simulink model "Three_Phase_SPWM_Boost_Rectifier2015b"  (Simulink 8.6)
settings: Solver=ode45  StartTime=0.0  StopTime=0.8  RelTol=1e-3
libraries: powerlib x20, simulink x4, powerlib_meascontrol x3
settings Model: Creator=sample  LastModifiedBy=A0109971
settings DebuggingCC: FcnCallInpInsideContextMsg=EnableAllAsWarning  AllowSymbolicDim=on

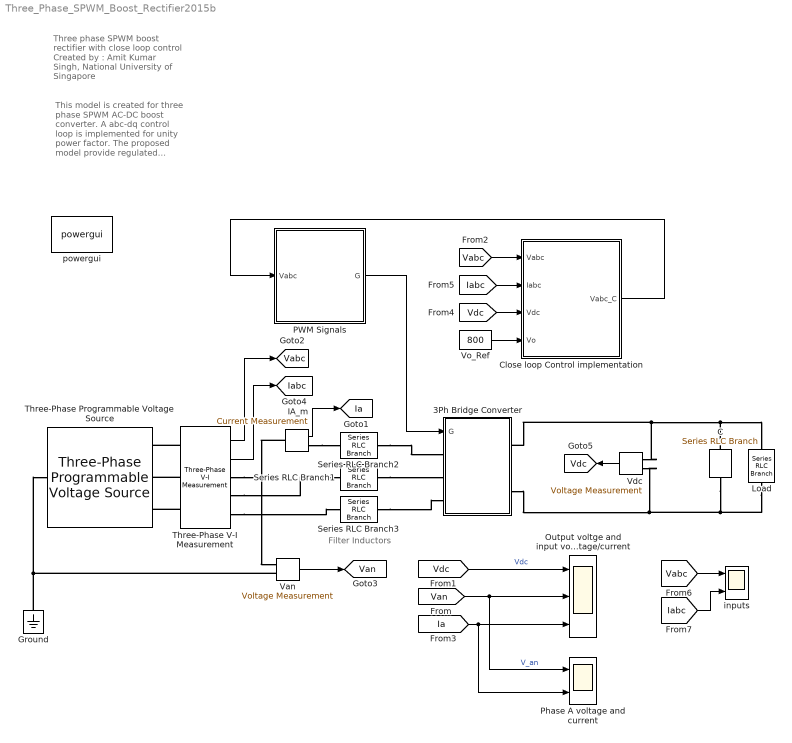
== system Three_Phase_SPWM_Boost_Rectifier2015b ==
  note: This model is created for three phase SPWM AC-DC boost converter. A abc-dq control loop is implemented for unity power factor. The proposed model provide
      | regulated output DC voltage with unity power factor and superior input power quality. The input voltage is three phase 230 V rms, 50 Hz. The output voltage is
      | 800 V DC.
  note: Three phase SPWM boost rectifier with close loop control
      |
      | Created by : Amit Kumar Singh, National University of Singapore
  note: Filter Inductors
  3Ph Bridge Converter : Subsystem
  C : powerlib/Elements/Series RLC Branch  LConnTagsString=__new0  RConnTagsString=__new0  BranchType=C  Resistance=1  Inductance=1e-3  SetiL0=off  InitialCurrent=0  Capacitance=1000e-6  Setx0=off  InitialVoltage=0  Measurements=None
  Close loop Control implementation : Subsystem
  Ground : powerlib/Elements/Ground  LConnTagsString=a
  IA_m : powerlib/Measurements/Current Measurement  PhasorSimulation=off  OutputType=Complex  PSBequivalent=0
  Load : powerlib/Elements/Series RLC Branch  LConnTagsString=__new0  RConnTagsString=__new0  BranchType=R  Resistance=10  Inductance=1e-3  SetiL0=off  InitialCurrent=0  Capacitance=0  Setx0=off  InitialVoltage=0  Measurements=None
  Output voltge and input voltage/current : Scope  NumInputPorts=3
  PWM Signals : Subsystem
  Phase A voltage and current : Scope  NumInputPorts=2
  Series RLC Branch1 : powerlib/Elements/Series RLC Branch  LConnTagsString=__new0  RConnTagsString=__new0  BranchType=RL  Resistance=.1  Inductance=1e-3  SetiL0=off  InitialCurrent=0  Capacitance=200e-6  Setx0=off  InitialVoltage=0  Measurements=None
  Series RLC Branch2 : powerlib/Elements/Series RLC Branch  LConnTagsString=__new0  RConnTagsString=__new0  BranchType=RL  Resistance=0.1  Inductance=1e-3  SetiL0=off  InitialCurrent=0  Capacitance=200e-6  Setx0=off  InitialVoltage=0  Measurements=None
  Series RLC Branch3 : powerlib/Elements/Series RLC Branch  LConnTagsString=__new0  RConnTagsString=__new0  BranchType=RL  Resistance=0.1  Inductance=1e-3  SetiL0=off  InitialCurrent=0  Capacitance=200e-6  Setx0=off  InitialVoltage=0  Measurements=None
  Three-Phase Programmable Voltage Source : powerlib/Electrical Sources/Three-Phase Programmable Voltage Source  PositiveSequence="[230*1.732  0 50]"  VariationEntity=None  VariationType=Table of time-amplitude pairs  VariationTypeAlt=Step  VariationStep=0.5  VariationRate=10  VariationMagnitude=0.3  VariationFrequency=2  VariationTiming=[1 2]  VariationPhaseA=off  Amplitudes=[1 0.8 1.2 1.0]  TimeValues=[0 0.1 0.15 0.2]  HarmonicGeneration=off  HarmonicA=[3 0.2 -25 0]  HarmonicB=[2 0.15 35 2]  Timing="[0.05  3]"  BusType=swing  Pref=0  Qref=0  Qmin=-inf  Qmax=inf
  Three-Phase V-I Measurement : powerlib/Measurements/Three-Phase V-I Measurement  VoltageMeasurement=phase-to-ground  SetLabelV=off  LabelV=Vabc  Vpu=off  VpuLL=off  CurrentMeasurement=yes  SetLabelI=off  LabelI=Iabc  Ipu=off  Pbase=100e6  Vbase=500e3  OutputType=Complex  PhasorSimulation=off  PSBequivalent=0
  Van : powerlib/Measurements/Voltage Measurement  Tag=PoWeRsYsTeMmEaSuReMeNt  PhasorSimulation=off  OutputType=Magnitude  PSBequivalent=0
  "Vdc " : powerlib/Measurements/Voltage Measurement  Tag=PoWeRsYsTeMmEaSuReMeNt  PhasorSimulation=off  OutputType=Magnitude  PSBequivalent=0
  Vo_Ref : Constant  Value=800
  inputs : Scope  NumInputPorts=2
  powergui : powerlib/powergui  Priority=1  SimulationMode=Discrete  SampleTime=2e-6  frequency=60  Iterations=50  frequencyindice=50  Pbase=100e6  ErrMax=1e-4  UnitsV=kV  UnitsW=MW  buscounter=0  FunctionMessages=off  echomessages=off  EnableUseOfTLC=off  CurrentSourceSwitches=off  DisableSnubberDevices=off  DisableRonSwitches=off  DisableVfSwitches=off  DisplayEquations=off  SolverType=Tustin  Interpol=off  ExternalGateDelay=off  methode=off  Ts=100  x0status=blocks  SPID=off  SwTol=0  HookPort=off  RestoreLinks=warning  ResistiveCurrentMeasurement=off  Frange=[0:2:500]  Ylog=off  Xlog=on  ShowGrid=off  save=off  variable=ZData  structure=ScopeData  ZoomFFT=off  StartTime=0.6  cycles=4  DisplayStyle=4  fundamental=50  FreqAxis=on  MaxFrequency=650  frequencyindicesteady=1  RmsSteady=1  display=off
  tag scope: Ia=global, Iabc=global, Vabc=global, Van=global, Vdc=global
  wires:
  [Van] -> Phase A voltage and current/1, Output voltge and input voltage/current/2  "V_an"
  "Vdc "/1 -> [Vdc]
  [Vdc] -> Output voltge and input voltage/current/1  "Vdc"
  Van/1 -> [Van]
  IA_m/1 -> [Ia]
  Three-Phase V-I Measurement/1 -> [Vabc]
  Three-Phase V-I Measurement/2 -> [Iabc]
  PWM Signals/1(G) -> 3Ph Bridge Converter/1(G)
  [Ia] -> Phase A voltage and current/2, Output voltge and input voltage/current/3
  [Vabc] -> Close loop Control implementation/1(Vabc)
  [Vdc] -> Close loop Control implementation/3(Vdc)
  [Iabc] -> Close loop Control implementation/2(Iabc)
  Close loop Control implementation/1(Vabc_C) -> PWM Signals/1(Vabc)
  [Vabc] -> inputs/1
  [Iabc] -> inputs/2
  Vo_Ref/1 -> Close loop Control implementation/4(Vo)
  connections:
  Load/RConn1 -- C/RConn1 -- "Vdc "/LConn2 -- 3Ph Bridge Converter/RConn2
  IA_m/LConn1 -- Three-Phase V-I Measurement/RConn1 -- Van/LConn1
  "Vdc "/LConn1 -- C/LConn1 -- Load/LConn1 -- 3Ph Bridge Converter/RConn1
  Series RLC Branch2/LConn1 -- 3Ph Bridge Converter/LConn1
  Series RLC Branch1/LConn1 -- 3Ph Bridge Converter/LConn2
  Series RLC Branch3/LConn1 -- 3Ph Bridge Converter/LConn3
  Van/LConn2 -- Three-Phase Programmable Voltage Source/LConn1 -- Ground/LConn1
  IA_m/RConn1 -- Series RLC Branch2/RConn1
  Three-Phase V-I Measurement/LConn1 -- Three-Phase Programmable Voltage Source/RConn1
  Three-Phase V-I Measurement/LConn2 -- Three-Phase Programmable Voltage Source/RConn2
  Three-Phase V-I Measurement/LConn3 -- Three-Phase Programmable Voltage Source/RConn3
  Three-Phase V-I Measurement/RConn2 -- Series RLC Branch1/RConn1
  Three-Phase V-I Measurement/RConn3 -- Series RLC Branch3/RConn1

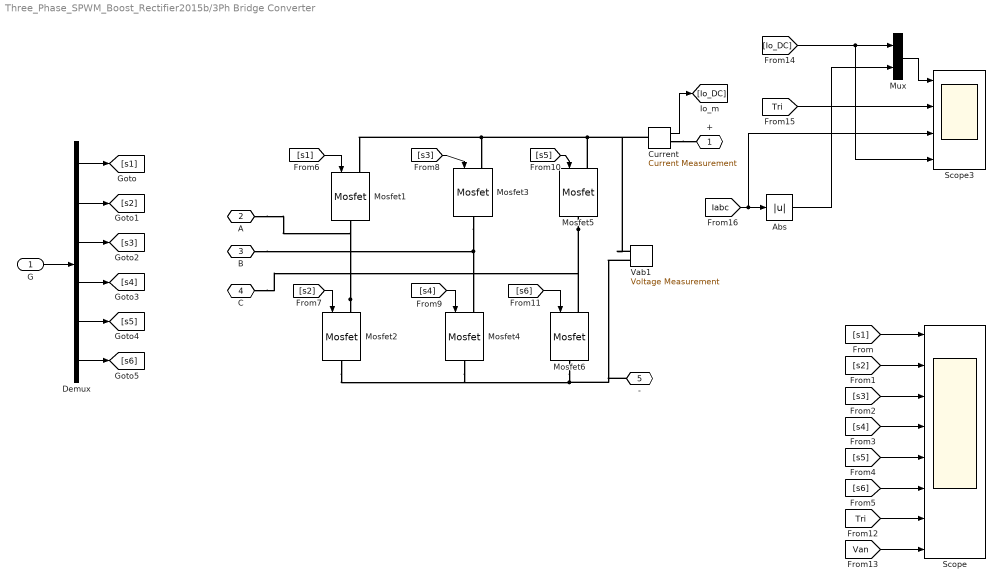
== system Three_Phase_SPWM_Boost_Rectifier2015b/3Ph Bridge Converter ==
  G : Inport
  Abs : Abs
  Current : powerlib/Measurements/Current Measurement  PhasorSimulation=off  OutputType=Complex  PSBequivalent=0
  Demux : Demux  Outputs=6
  Mosfet{1..6} (6 alike) : powerlib/Power Electronics/Mosfet  Ron=0.1  Lon=0  Rd=0.01  Vfd=0  IC=0  Rs=1e5  Cs=inf  Measurements=off
  Mux : Mux  Inputs=2
  Scope : Scope  NumInputPorts=8
  Scope3 : Scope  NumInputPorts=4
  Vab1 : powerlib/Measurements/Voltage Measurement  Tag=PoWeRsYsTeMmEaSuReMeNt  PhasorSimulation=off  OutputType=Magnitude  PSBequivalent=0
  + : PMIOPort  Port=1  Side=Right
  A : PMIOPort  Port=2  Side=Left
  B : PMIOPort  Port=3  Side=Left
  C : PMIOPort  Port=4  Side=Left
  - : PMIOPort  Port=5  Side=Right
  wires:
  [s1] -> Mosfet1/1
  [s2] -> Mosfet2/1
  [s3] -> Mosfet3/1
  [s4] -> Mosfet4/1
  [s5] -> Mosfet5/1
  [s6] -> Mosfet6/1
  Demux/1 -> [s1]
  Demux/2 -> [s2]
  Demux/3 -> [s3]
  Demux/4 -> [s4]
  Demux/5 -> [s5]
  Demux/6 -> [s6]
  G/1 -> Demux/1
  Current/1 -> [Io_DC]
  [s1] -> Scope/1
  [s2] -> Scope/2
  [s3] -> Scope/3
  [s4] -> Scope/4
  [s5] -> Scope/5
  [s6] -> Scope/6
  [Tri] -> Scope/7
  [Van] -> Scope/8
  [Tri] -> Scope3/2
  [Io_DC] -> Scope3/4, Mux/1
  Mux/1 -> Scope3/1
  [Iabc] -> Scope3/3, Abs/1
  Abs/1 -> Mux/2
  connections:
  Mosfet5/LConn1 -- Vab1/LConn1 -- Current/LConn1 -- Mosfet1/LConn1 -- Mosfet3/LConn1
  Mosfet6/RConn1 -- Vab1/LConn2 -- -/RConn1 -- Mosfet2/RConn1 -- Mosfet4/RConn1
  Mosfet2/LConn1 -- Mosfet1/RConn1 -- A/RConn1
  Mosfet3/RConn1 -- Mosfet4/LConn1 -- B/RConn1
  Mosfet5/RConn1 -- Mosfet6/LConn1 -- C/RConn1
  Current/RConn1 -- +/RConn1

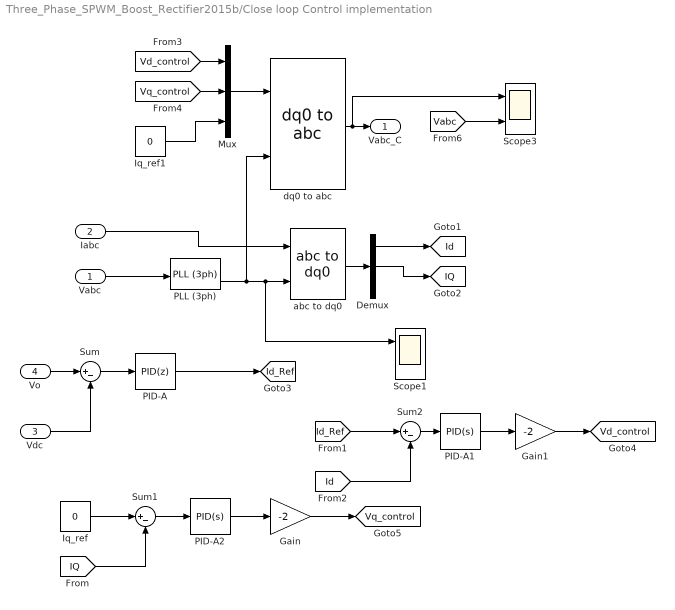
== system Three_Phase_SPWM_Boost_Rectifier2015b/Close loop Control implementation ==
  Vabc : Inport
  Iabc : Inport  Port=2
  Vdc : Inport  Port=3
  Vo : Inport  Port=4
  Demux : Demux  Outputs=3
  Gain : Gain  Gain=-2
  Gain1 : Gain  Gain=-2
  Iq_ref : Constant  Value=0
  Iq_ref1 : Constant  Value=0
  Mux : Mux  Inputs=3
  PID-A : simulink/Continuous/PID Controller  Controller=PID  TimeDomain=Discrete-time  SampleTime=2e-6  IntegratorMethod=Forward Euler  FilterMethod=Forward Euler  Form=Parallel  UseFilter=on  ControllerParametersSource=internal  P=0.2  I=0.2/0.002  D=0  N=100  InitialConditionSource=internal  InitialConditionForIntegrator=0  InitialConditionForFilter=0  ExternalReset=none  LimitOutput=off  UpperSaturationLimit=inf  LowerSaturationLimit=-inf  LinearizeAsGain=on  AntiWindupMode=none  Kb=1  TrackingMode=off  Kt=1  PParamMin=[]  PParamMax=[]  IParamMin=[]  IParamMax=[]  DParamMin=[]  DParamMax=[]  NParamMin=[]  NParamMax=[]  KbParamMin=[]  KbParamMax=[]  KtParamMin=[]  KtParamMax=[]  POutMin=[]  POutMax=[]  IOutMin=[]  IOutMax=[]  DOutMin=[]  DOutMax=[]  NOutMin=[]  NOutMax=[]  KbOutMin=[]  KbOutMax=[]  KtOutMin=[]  KtOutMax=[]  IntegratorOutMin=[]  IntegratorOutMax=[]  FilterOutMin=[]  FilterOutMax=[]  SumOutMin=[]  SumOutMax=[]  SumI1OutMin=[]  SumI1OutMax=[]  SumI2OutMin=[]  SumI2OutMax=[]  SumI3OutMin=[]  SumI3OutMax=[]  SumDOutMin=[]  SumDOutMax=[]  SaturationOutMin=[]  SaturationOutMax=[]  IntegratorContinuousStateAttributes=''  IntegratorStateMustResolveToSignalObject=off  IntegratorRTWStateStorageClass=Auto  FilterContinuousStateAttributes=''  FilterStateMustResolveToSignalObject=off  FilterRTWStateStorageClass=Auto  DifferentiatorICPrevScaledInput=0  DifferentiatorOutMin=[]  DifferentiatorOutMax=[]
  PID-A1 : simulink/Continuous/PID Controller  Controller=PID  TimeDomain=Continuous-time  SampleTime=-1  IntegratorMethod=Forward Euler  FilterMethod=Forward Euler  Form=Parallel  UseFilter=on  ControllerParametersSource=internal  P=6.225/270  I=0.0231/1.172e-3  D=0  N=100  InitialConditionSource=internal  InitialConditionForIntegrator=0  InitialConditionForFilter=0  ExternalReset=none  LimitOutput=off  UpperSaturationLimit=inf  LowerSaturationLimit=-inf  LinearizeAsGain=on  AntiWindupMode=none  Kb=1  TrackingMode=off  Kt=1  PParamMin=[]  PParamMax=[]  IParamMin=[]  IParamMax=[]  DParamMin=[]  DParamMax=[]  NParamMin=[]  NParamMax=[]  KbParamMin=[]  KbParamMax=[]  KtParamMin=[]  KtParamMax=[]  POutMin=[]  POutMax=[]  IOutMin=[]  IOutMax=[]  DOutMin=[]  DOutMax=[]  NOutMin=[]  NOutMax=[]  KbOutMin=[]  KbOutMax=[]  KtOutMin=[]  KtOutMax=[]  IntegratorOutMin=[]  IntegratorOutMax=[]  FilterOutMin=[]  FilterOutMax=[]  SumOutMin=[]  SumOutMax=[]  SumI1OutMin=[]  SumI1OutMax=[]  SumI2OutMin=[]  SumI2OutMax=[]  SumI3OutMin=[]  SumI3OutMax=[]  SumDOutMin=[]  SumDOutMax=[]  SaturationOutMin=[]  SaturationOutMax=[]  IntegratorContinuousStateAttributes=''  IntegratorStateMustResolveToSignalObject=off  IntegratorRTWStateStorageClass=Auto  FilterContinuousStateAttributes=''  FilterStateMustResolveToSignalObject=off  FilterRTWStateStorageClass=Auto  DifferentiatorICPrevScaledInput=0  DifferentiatorOutMin=[]  DifferentiatorOutMax=[]
  PID-A2 : simulink/Continuous/PID Controller  Controller=PID  TimeDomain=Continuous-time  SampleTime=-1  IntegratorMethod=Forward Euler  FilterMethod=Forward Euler  Form=Parallel  UseFilter=on  ControllerParametersSource=internal  P=6.225/270  I=0.0231/1.172e-3  D=0  N=100  InitialConditionSource=internal  InitialConditionForIntegrator=0  InitialConditionForFilter=0  ExternalReset=none  LimitOutput=off  UpperSaturationLimit=inf  LowerSaturationLimit=-inf  LinearizeAsGain=on  AntiWindupMode=none  Kb=1  TrackingMode=off  Kt=1  PParamMin=[]  PParamMax=[]  IParamMin=[]  IParamMax=[]  DParamMin=[]  DParamMax=[]  NParamMin=[]  NParamMax=[]  KbParamMin=[]  KbParamMax=[]  KtParamMin=[]  KtParamMax=[]  POutMin=[]  POutMax=[]  IOutMin=[]  IOutMax=[]  DOutMin=[]  DOutMax=[]  NOutMin=[]  NOutMax=[]  KbOutMin=[]  KbOutMax=[]  KtOutMin=[]  KtOutMax=[]  IntegratorOutMin=[]  IntegratorOutMax=[]  FilterOutMin=[]  FilterOutMax=[]  SumOutMin=[]  SumOutMax=[]  SumI1OutMin=[]  SumI1OutMax=[]  SumI2OutMin=[]  SumI2OutMax=[]  SumI3OutMin=[]  SumI3OutMax=[]  SumDOutMin=[]  SumDOutMax=[]  SaturationOutMin=[]  SaturationOutMax=[]  IntegratorContinuousStateAttributes=''  IntegratorStateMustResolveToSignalObject=off  IntegratorRTWStateStorageClass=Auto  FilterContinuousStateAttributes=''  FilterStateMustResolveToSignalObject=off  FilterRTWStateStorageClass=Auto  DifferentiatorICPrevScaledInput=0  DifferentiatorOutMin=[]  DifferentiatorOutMax=[]
  PLL (3ph) : powerlib_meascontrol/PLL/PLL (3ph)  Fmin=45  Par_Init=[0, 60]  ParK=[180, 3200, 1]  TcD=1e-4  MaxRateChangeFreq=12  FilterCutOffFreq=25  Ts=0  AGC=on
  Scope1 : Scope  NumInputPorts=2
  Scope3 : Scope  NumInputPorts=2
  Sum : Sum  Inputs=|+-
  Sum1 : Sum  Inputs=|+-
  Sum2 : Sum  Inputs=|+-
  abc to dq0 : powerlib_meascontrol/Transformations/abc to dq0  Alignment=90 degrees behind phase A axis
  dq0 to abc : powerlib_meascontrol/Transformations/dq0 to abc  Alignment=90 degrees behind phase A axis
  Vabc_C : Outport
  tag scope: IQ=global, Id=global, Id_Ref=global, Vd_control=global, Vq_control=global
  wires:
  Vabc/1 -> PLL (3ph)/1
  PLL (3ph)/2 -> dq0 to abc/2, Scope1/1, abc to dq0/2
  Iabc/1 -> abc to dq0/1
  abc to dq0/1 -> Demux/1
  Demux/1 -> [Id]
  Demux/2 -> [IQ]
  Iq_ref/1 -> Sum1/1
  [IQ] -> Sum1/2
  Sum1/1 -> PID-A2/1
  [Id_Ref] -> Sum2/1
  [Id] -> Sum2/2
  Sum2/1 -> PID-A1/1
  PID-A2/1 -> Gain/1
  PID-A1/1 -> Gain1/1
  Mux/1 -> dq0 to abc/1
  [Vd_control] -> Mux/1
  [Vq_control] -> Mux/2
  Iq_ref1/1 -> Mux/3
  dq0 to abc/1 -> Scope3/1, Vabc_C/1
  Gain/1 -> [Vq_control]
  Gain1/1 -> [Vd_control]
  [Vabc] -> Scope3/2
  Sum/1 -> PID-A/1
  Vo/1 -> Sum/1
  Vdc/1 -> Sum/2
  PID-A/1 -> [Id_Ref]

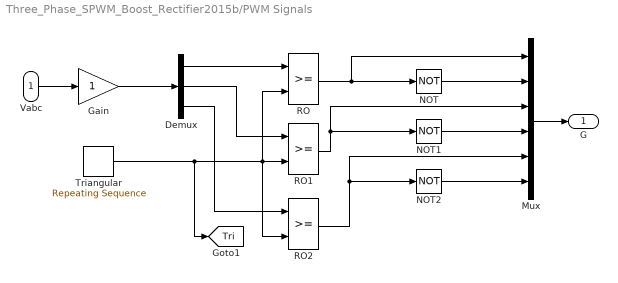
== system Three_Phase_SPWM_Boost_Rectifier2015b/PWM Signals ==
  Vabc : Inport
  Demux : Demux  Outputs=3
  Gain : Gain
  Mux : Mux  Inputs=6
  NOT : Logic  Operator=NOT  IconShape=distinctive  AllPortsSameDT=off  OutDataTypeStr=boolean
  NOT1 : Logic  Operator=NOT  IconShape=distinctive  AllPortsSameDT=off  OutDataTypeStr=boolean
  NOT2 : Logic  Operator=NOT  IconShape=distinctive  AllPortsSameDT=off  OutDataTypeStr=boolean
  RO : RelationalOperator  OutDataTypeStr=boolean
  RO1 : RelationalOperator  OutDataTypeStr=boolean
  RO2 : RelationalOperator  OutDataTypeStr=boolean
  Triangular : simulink/Sources/Repeating Sequence  rep_seq_t="[0  1/(10e3) 1/(5e3) ]"  rep_seq_y=[-1 1 -1 ]
  G : Outport
  tag scope: Tri=global
  wires:
  Vabc/1 -> Gain/1
  Gain/1 -> Demux/1
  Demux/1 -> RO/1
  Demux/2 -> RO1/1
  Demux/3 -> RO2/1
  Triangular/1 -> [Tri], RO1/2, RO/2, RO2/2
  RO/1 -> Mux/1, NOT/1
  NOT/1 -> Mux/2
  RO2/1 -> NOT2/1, Mux/5
  RO1/1 -> NOT1/1, Mux/3
  NOT1/1 -> Mux/4
  NOT2/1 -> Mux/6
  Mux/1 -> G/1
